simulink model "SimulationSansObservateur"  (R2017a)
settings: Solver=ode14x  StartTime=1  StopTime=Ts  FixedStep=0.01  RelTol=1e-3
values from neighbouring files (symbols this model uses):
  bornes = [minn, maxx]    [Model.m]
  Choix = -1    [Data.m]
  dmin = 5    [Distance_Securite_Vitesse.m]    (also in Model.m)
  K1 = cat(3,K1(1:r).sys)    [Mainscript.m]
  M = inv(X)    [Gainfind.m]    (also in GainfindV2.m; GainfindVTD.m; Mainscript.m = cat(3,M(1:r).sys); Observateurflou.m = inv(P))
  Parametres = [ax, bx, Rap, alpha, tau]    [Model.m]
  Parametres2 = [tr, f]    [Model.m]
  Pt0 = 50    [Data.m]
  Vt0 = 23.946459624338537    (= 23.9464596243)    [Data.m]
libraries: simulink x2
settings Model: SimulationMode=accelerator  Creator=MONCEF  LastModifiedBy=MONCEF

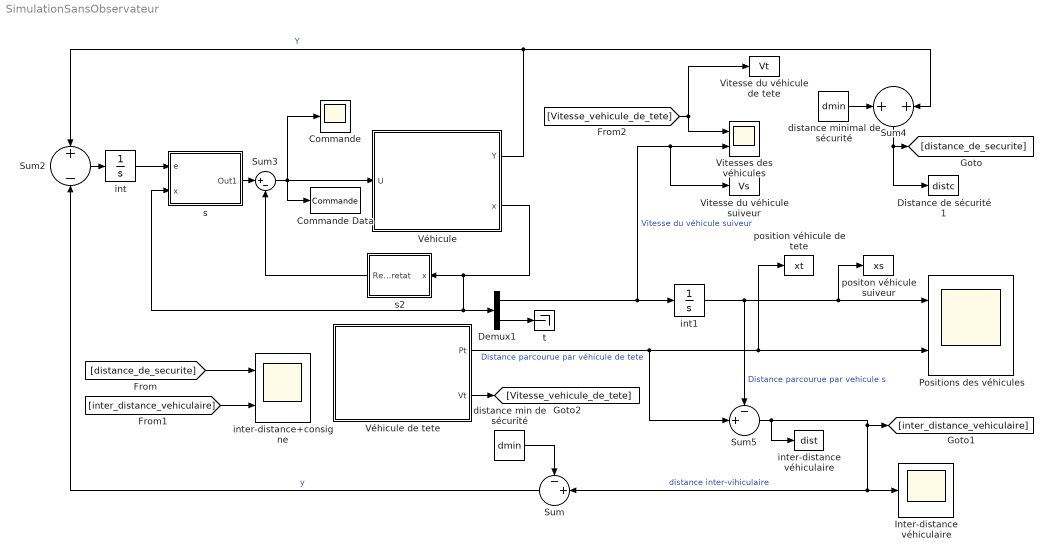
== system SimulationSansObservateur ==
  " Vitesses des véhicules" : Scope  NumInputPorts=2
  Commande : Scope
  Commande Data : ToWorkspace  VariableName=Commande  SaveFormat=Structure With Time  SampleTime=0.1
  Demux1 : Demux  Outputs=2
  Distance de sécurité 1 : ToWorkspace  VariableName=distc  SaveFormat=Structure With Time  SampleTime=0.1
  Inter-distance véhiculaire : Scope
  Positions des véhicules : Scope  NumInputPorts=2
  Sum : Sum  Inputs=-+|
  Sum2 : Sum  Inputs=+|-
  Sum3 : Sum  Inputs=|+-
  Sum4 : Sum  Inputs=+|+
  Sum5 : Sum  Inputs=-+|
  Vitesse du véhicule de tete : ToWorkspace  VariableName=Vt  SaveFormat=Structure With Time  SampleTime=0.1
  Vitesse du véhicule suiveur : ToWorkspace  VariableName=Vs  SaveFormat=Structure With Time  SampleTime=0.1
  Véhicule : Subsystem
      mask Display: image(fullfile(pwd,'Images','VehiculeSuiveur.jpg'));
  Véhicule de tete : Subsystem
      mask Display: image(fullfile(pwd,'Images','VehiculeTete.png'));
  "distance min de sécurité " : Constant  Value=dmin
  distance minimal de sécurité : Constant  Value=dmin
  int : Integrator
      mask Display: image(fullfile(pwd,'Images','Integrateur.png'));
  int1 : Integrator
      mask Display: image(fullfile(pwd,'Images','Integrateur.png'));
  "inter-distance véhiculaire " : ToWorkspace  VariableName=dist  SaveFormat=Structure With Time  SampleTime=0.1
  inter-distance+consigne : Scope  NumInputPorts=2
  position véhicule de tete : ToWorkspace  VariableName=xt  SaveFormat=Structure With Time  SampleTime=0.1
  positon véhicule suiveur : ToWorkspace  VariableName=xs  SaveFormat=Structure With Time  SampleTime=0.1
  s : Subsystem
      mask Display: image(fullfile(pwd,'Images','Gain_d_integ.png'));
  s2 : Subsystem
      mask Display: image(fullfile(pwd,'Images','Retour d''état.png'));
  t : Terminator
  wires:
  [Vitesse_vehicule_de_tete] -> Vitesse du véhicule de tete/1, " Vitesses des véhicules"/1
  Véhicule de tete/1(Pt) -> Sum5/2, Positions des véhicules/2, position véhicule de tete/1  "Distance parcourue par véhicule de tete"
  distance minimal de sécurité/1 -> Sum4/1
  Véhicule/1(Y) -> Sum4/2, Sum2/1  "Y"
  Demux1/1 -> int1/1, " Vitesses des véhicules"/2, Vitesse du véhicule suiveur/1  "Vitesse du véhicule suiveur"
  "distance min de sécurité "/1 -> Sum/1
  Sum/1 -> Sum2/2  "y"
  Demux1/2 -> t/1
  s2/1(Retouretat) -> Sum3/2
  Véhicule/2(x) -> s/2(x), Demux1/1, s2/1(x)
  int1/1 -> Sum5/1, Positions des véhicules/1, positon véhicule suiveur/1  "Distance parcourue par vehicule s"
  Sum4/1 -> [distance_de_securite], Distance de sécurité 1/1
  Sum5/1 -> "inter-distance véhiculaire "/1, Sum/2, Inter-distance véhiculaire/1, [inter_distance_vehiculaire]  "distance inter-vihiculaire"
  Sum2/1 -> int/1
  s/1(Out1) -> Sum3/1
  int/1 -> s/1(e)
  Sum3/1 -> Commande/1, Véhicule/1(U), Commande Data/1
  [distance_de_securite] -> inter-distance+consigne/1
  [inter_distance_vehiculaire] -> inter-distance+consigne/2
  Véhicule de tete/2(Vt) -> [Vitesse_vehicule_de_tete]

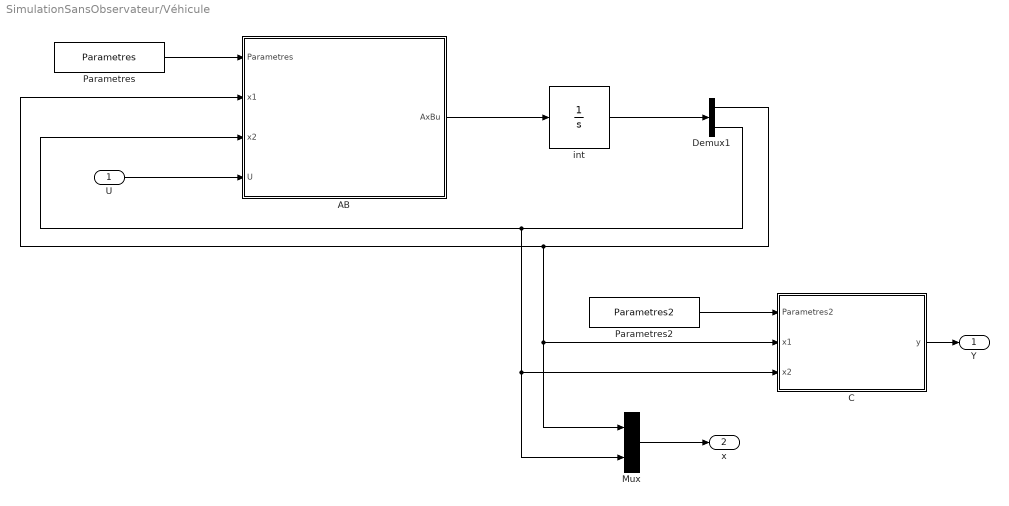
== system SimulationSansObservateur/Véhicule ==
  U : Inport
  AB : MATLAB Function  TreatAsAtomicUnit=on
  C : MATLAB Function  TreatAsAtomicUnit=on
  Demux1 : Demux  Outputs=2
  Mux : Mux  Inputs=2
  Parametres : Constant  Value=Parametres
  Parametres2 : Constant  Value=Parametres2
  int : Integrator
      mask Display: image(fullfile(pwd,'Images','Integrateur.png'));
  Y : Outport
  x : Outport  Port=2
  wires:
  C/1(y) -> Y/1
  Parametres/1 -> AB/1(Parametres)
  Parametres2/1 -> C/1(Parametres2)
  U/1 -> AB/4(U)
  AB/1(AxBu) -> int/1
  Demux1/2 -> Mux/2, C/3(x2), AB/3(x2)
  Demux1/1 -> Mux/1, C/2(x1), AB/2(x1)
  Mux/1 -> x/1
  int/1 -> Demux1/1

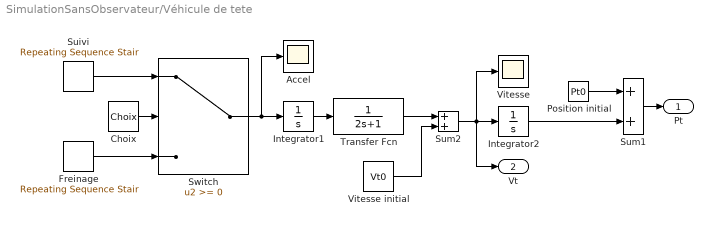
== system SimulationSansObservateur/Véhicule de tete ==
  Accel : Scope
  Choix : Constant  Value=Choix
  Freinage : simulink/Sources/Repeating Sequence Stair  OutValues=[0 0-3 0 0 0 0].'  tsamp=8  OutMin=[]  OutMax=[]  OutDataTypeStr=double  OutputDataTypeScalingMode=double  OutDataType=fixdt(0,8)  ConRadixGroup=Best Precision: Vector-wise  OutScaling=2^-12
  Integrator1 : Integrator
  Integrator2 : Integrator
  Position initial : Constant  Value=Pt0
  Suivi : simulink/Sources/Repeating Sequence Stair  OutValues="[1 1 0 0 -0.375 0 0 -0.375 0 0 0.25  0 0 -0.75 0 -0.75].'"  tsamp=10  OutMin=[]  OutMax=[]  OutDataTypeStr=double  OutputDataTypeScalingMode=double  OutDataType=fixdt(0,8)  ConRadixGroup=Best Precision: Vector-wise  OutScaling=2^-12
  Sum1 : Sum
  Sum2 : Sum
  Switch : Switch
  Transfer Fcn : TransferFcn  Denominator=[2 1]
  Vitesse : Scope
  Vitesse initial : Constant  Value=Vt0
  Pt : Outport
  Vt : Outport  Port=2
  wires:
  Vitesse initial/1 -> Sum2/2
  Transfer Fcn/1 -> Sum2/1
  Integrator1/1 -> Transfer Fcn/1
  Integrator2/1 -> Sum1/2
  Position initial/1 -> Sum1/1
  Sum1/1 -> Pt/1
  Sum2/1 -> Integrator2/1, Vitesse/1, Vt/1
  Switch/1 -> Integrator1/1, Accel/1
  Suivi/1 -> Switch/1
  Freinage/1 -> Switch/3
  Choix/1 -> Switch/2

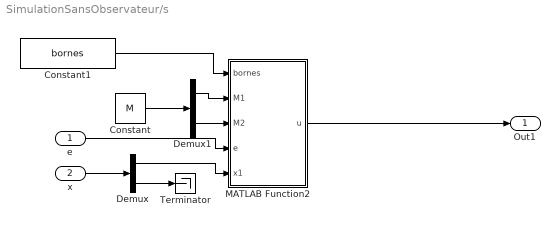
== system SimulationSansObservateur/s ==
  e : Inport
  x : Inport  Port=2
  Constant : Constant  Value=M
  Constant1 : Constant  Value=bornes
  Demux : Demux  Outputs=2
  Demux1 : Demux  Outputs=2
  MATLAB Function2 : MATLAB Function  TreatAsAtomicUnit=on
  Terminator : Terminator
  Out1 : Outport
  wires:
  MATLAB Function2/1(u) -> Out1/1
  e/1 -> MATLAB Function2/4(e)
  x/1 -> Demux/1
  Demux/1 -> MATLAB Function2/5(x1)
  Demux/2 -> Terminator/1
  Constant/1 -> Demux1/1
  Demux1/1 -> MATLAB Function2/2(M1)
  Demux1/2 -> MATLAB Function2/3(M2)
  Constant1/1 -> MATLAB Function2/1(bornes)

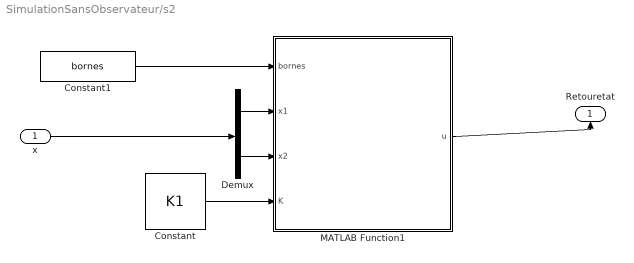
== system SimulationSansObservateur/s2 ==
  x : Inport
  Constant : Constant  Value=K1
  Constant1 : Constant  Value=bornes
  Demux : Demux  Outputs=2
  MATLAB Function1 : MATLAB Function  TreatAsAtomicUnit=on
  Retouretat : Outport
  wires:
  Constant/1 -> MATLAB Function1/4(K)
  x/1 -> Demux/1
  Demux/2 -> MATLAB Function1/3(x2)
  Demux/1 -> MATLAB Function1/2(x1)
  MATLAB Function1/1(u) -> Retouretat/1
  Constant1/1 -> MATLAB Function1/1(bornes)

== matlab function SimulationSansObservateur/s2/MATLAB Function1 ==
  data: bornes input; x1 input; x2 input; u output; K input
function u = fcn(bornes,x1,x2,K)

x=[x1;x2];

K1=K(:,:,1);
K2=K(:,:,2);

min = bornes(1);
max = bornes(2);
T1=(x1-min)/(max-min);
T2=(max-x1)/(max-min);



u =(T1*K1+T2*K2)*x;

== matlab function SimulationSansObservateur/s/MATLAB Function2 ==
  data: bornes input; M1 input; M2 input; e input; u output; x1 input
function u = fcn(bornes,M1,M2,e,x1)

min = bornes(1);
max = bornes(2);
T1=(x1-min)/(max-min);
T2=(max-x1)/(max-min);

u =(T1*M1+T2*M2)*e;

== matlab function SimulationSansObservateur/Véhicule/AB ==
  data: Parametres input; x1 input; AxBu output; x2 input; U input
function AxBu = fcn(Parametres,x1,x2,U)

ax = Parametres(1);
bx = Parametres(2);
Rap = Parametres(3);
alpha = Parametres(4);
tau = Parametres(5);

%define the systeme matrix
A =[-(ax+bx*x1)/alpha Rap/alpha; 0 -1/tau];
B =[0 ; 1/tau];



AxBu = A*[x1;x2]+B*U;

== matlab function SimulationSansObservateur/Véhicule/C ==
  data: Parametres2 input; x1 input; y output; x2 input
function y = fcn(Parametres2,x1,x2)
tr = Parametres2(1);
f = Parametres2(2);

C = [tr+f*x1 0];
y =C*[x1;x2];
